simulink model "tensegrity_Val_like_sim"  (R2022b)
settings: Solver=VariableStepAuto  StartTime=0.0  StopTime=10.0  MaxStep=0.01  RelTol=1e-3
values from neighbouring files (symbols this model uses):
  a = 0.015    [parameters.m]
  bar_or_cable = 1    [parameters.m]
  bb = 1    [parameters.m]
  F1 = [pos1(1), pos1(2), pos1(3)]    [parameters.m]
  F2 = [pos1(1)+dist, pos1(2), pos1(3)]    [parameters.m]
  F3 = [pos1(1)+dist/2, pos1(2)+dist, pos1(3)]    [parameters.m]
  F4 = [pos2(1), pos2(2), pos2(3)]    [parameters.m]
  F5 = [pos2(1)+dist, pos2(2), pos2(3)]    [parameters.m]
  F6 = [pos2(1)+dist/2, pos2(2)+dist, pos2(3)]    [parameters.m]
  F7 = [pos3(1), pos3(2), pos3(3)]    [parameters.m]
  F8 = [pos3(1)+dist, pos3(2), pos3(3)]    [parameters.m]
  F9 = [pos3(1)+dist/2, pos3(2)+dist, pos3(3)]    [parameters.m]
  kk = 500    [parameters.m]
  l = [0.08 0.08 0.08 0.15]'    [parameters.m]
  lengths_0 = [lengths_0; l_i]    [tensegrity_Val_like.m]
  lf = 0.05*ones(9, 1)    [parameters.m]
undefined symbols (not defined in the file or in its folder): X, Y, Z
libraries: sm_lib x33, nesl_utility x31
settings Model: Creator=zavrel  LastModifiedBy=zavrel

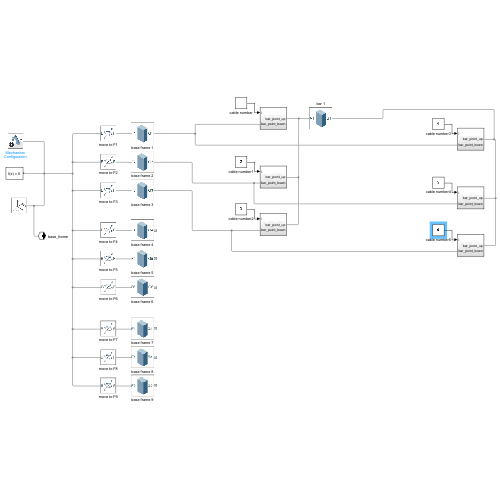
[thumbnail: Simulink's stored preview of the top-level diagram]
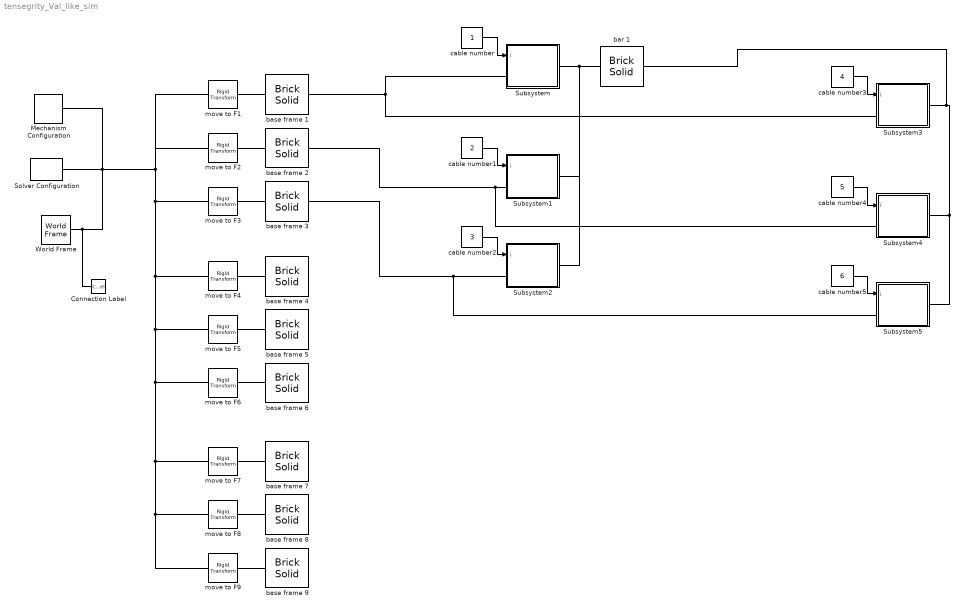
== system tensegrity_Val_like_sim ==
  Connection Label : ConnectionLabel  Label=base_frame
  Mechanism Configuration : sm_lib/Utilities/Mechanism Configuration  UniformGravity=Constant  GravityVector=[0 0 -9.80665]  GravityUnits=m/s^2  LinearizationDelta=0.001  JointModeTransitionNonlinearIterations=2
  Solver Configuration : nesl_utility/Solver Configuration  PhysicalDomain=network_engine_domain  SubClassName=solver  LeftPortType=input  RightPortType=generic  Tones=[]  Harmonics=[]  SimulateNoise=off  Profile=off  UseLocalSampling=off  EnableSwitchedLinearOptims=on  FrequencyDomain=off  UseCCode=off  RelTol=0.001  AbsTol=0.001  MinStep=1e-09  ToWorkspace=off  RevertToSquareIcSolve=off  NumHomotopyIterations=100  PhasorMode=off  PhasorModeNumHarmonics=1  ConsistencySolver=NEWTON_XTOL_AFTER_FTOL  IndexReductionMethod=DerivativeReplacement  DoDC=off  ResidualTolerance=1e-09  ConsistencyTolSource=GLOBAL  ConsistencyAbsTol=0.001  ConsistencyRelTol=0.001  ConsistencyTolFactor=0.001  UseLocalSolver=off  LocalSolverChoice=NE_BACKWARD_EULER_ADVANCER  ResolveIndetEquations=on  FunctionEvalNumThread=1  LocalSolverSampleTime=0.001  DoFixedCost=off  MaxNonlinIter=3  MaxModeIter=2  ComputeImpulses=off  ImpulseIterations=2  LinearAlgebra=auto  LinearAlgebraNumThread=0  EquationFormulation=NE_TIME_EF  DelaysMemoryBudget=1024  AutomaticFiltering=on  FilteringTimeConstant=0.001  PartitionStorageMethod=AS_NEEDED  PartitionMemoryBudget=1024  PartitionMethod=ROBUST
  Subsystem : Subsystem
  Subsystem1 : Subsystem
  Subsystem2 : Subsystem
  Subsystem3 : Subsystem
  Subsystem4 : Subsystem
  Subsystem5 : Subsystem
  World Frame : sm_lib/Frames and Transforms/World Frame
  bar 1 : sm_lib/Body Elements/Brick Solid  GraphicAmbientColor=[0.15 0.15 0.15 1.0]  BasedOnType=Density  BrickDimensions=[a a l(1)]  BrickDimensionUnits=m  CenterOfMass=[0 0 0]  CenterOfMassUnits=m  GraphicDiffuseColor=[0.5 0.5 0.5]  Density=rho  DensityUnits=kg/m^3  DoExposeReferenceFrame=off  GraphicEmissiveColor=[0.0 0.0 0.0 1.0]  ExportEntireGeometry=off  SerializedFrames=<Frames><Frame><Id>Frame1</Id><Value><Name>A1</Name><Origin><Source>GeometricFeature</Source><FeatureName>-z surface</FeatureName></Origin><PrimaryAxis><DefinedDirection>+Z</DefinedDirection><Source>ReferenceFrame</Source><SourceDirection>+Z</SourceDirection><FeatureName></FeatureName></PrimaryAxis><SecondaryAxis><DefinedDirection>+X</DefinedDirection><Source>ReferenceFrame</Source><SourceDirection>+X</SourceDirection><FeatureName></FeatureName></SecondaryAxis></Value></Frame><Frame><Id>Frame2</Id><Value><Name>B1</Name><Origin><Source>GeometricFeature</Source><FeatureName>+z surface</FeatureName></Origin><PrimaryAxis><DefinedDirection>+Z</DefinedDirection><Source>ReferenceFrame</Source><SourceDirection>+Z</SourceDirection><FeatureName></FeatureName></PrimaryAxis><SecondaryAxis><DefinedDirection>+X</DefinedDirection><Source>ReferenceFrame</Source><SourceDirection>+X</SourceDirection><FeatureName></FeatureName></SecondaryAxis></Value></Frame></Frames>  MarkerShape=Sphere  MarkerSize=10  GraphicType=FromGeometry  InertiaType=CalculateFromGeometry  Mass=1  MassUnits=kg  MomentsOfInertia=[1 1 1]  MomentsOfInertiaUnits=kg*m^2  GraphicOpacity=1.0  ProductsOfInertia=[0 0 0]  ProductsOfInertiaUnits=kg*m^2  GraphicShininess=75  GraphicSpecularColor=[0.5 0.5 0.5 1.0]  GraphicVisPropType=SimpleVisualProperties
  base frame 1 : sm_lib/Body Elements/Brick Solid  GraphicAmbientColor=[0.15 0.15 0.15 1.0]  BasedOnType=Density  BrickDimensions=[a a lf(1)]  BrickDimensionUnits=m  CenterOfMass=[0 0 0]  CenterOfMassUnits=m  GraphicDiffuseColor=[0.5 0.5 0.5]  Density=rho  DensityUnits=kg/m^3  DoExposeReferenceFrame=off  GraphicEmissiveColor=[0.0 0.0 0.0 1.0]  ExportEntireGeometry=off  SerializedFrames=<Frames><Frame><Id>Frame1</Id><Value><Name>F1</Name><Origin><Source>GeometricFeature</Source><FeatureName>-z surface</FeatureName></Origin><PrimaryAxis><DefinedDirection>+Z</DefinedDirection><Source>ReferenceFrame</Source><SourceDirection>+Z</SourceDirection><FeatureName></FeatureName></PrimaryAxis><SecondaryAxis><DefinedDirection>+X</DefinedDirection><Source>ReferenceFrame</Source><SourceDirection>+X</SourceDirection><FeatureName></FeatureName></SecondaryAxis></Value></Frame><Frame><Id>Frame2</Id><Value><Name>G1</Name><Origin><Source>GeometricFeature</Source><FeatureName>+z surface</FeatureName></Origin><PrimaryAxis><DefinedDirection>+Z</DefinedDirection><Source>ReferenceFrame</Source><SourceDirection>+Z</SourceDirection><FeatureName></FeatureName></PrimaryAxis><SecondaryAxis><DefinedDirection>+X</DefinedDirection><Source>ReferenceFrame</Source><SourceDirection>+X</SourceDirection><FeatureName></FeatureName></SecondaryAxis></Value></Frame></Frames>  MarkerShape=Sphere  MarkerSize=10  GraphicType=FromGeometry  InertiaType=CalculateFromGeometry  Mass=1  MassUnits=kg  MomentsOfInertia=[1 1 1]  MomentsOfInertiaUnits=kg*m^2  GraphicOpacity=1.0  ProductsOfInertia=[0 0 0]  ProductsOfInertiaUnits=kg*m^2  GraphicShininess=75  GraphicSpecularColor=[0.5 0.5 0.5 1.0]  GraphicVisPropType=SimpleVisualProperties
  base frame 2 : sm_lib/Body Elements/Brick Solid  GraphicAmbientColor=[0.15 0.15 0.15 1.0]  BasedOnType=Density  BrickDimensions=[a a lf(2)]  BrickDimensionUnits=m  CenterOfMass=[0 0 0]  CenterOfMassUnits=m  GraphicDiffuseColor=[0.5 0.5 0.5]  Density=rho  DensityUnits=kg/m^3  DoExposeReferenceFrame=off  GraphicEmissiveColor=[0.0 0.0 0.0 1.0]  ExportEntireGeometry=off  SerializedFrames=<Frames><Frame><Id>Frame1</Id><Value><Name>F2</Name><Origin><Source>GeometricFeature</Source><FeatureName>-z surface</FeatureName></Origin><PrimaryAxis><DefinedDirection>+Z</DefinedDirection><Source>ReferenceFrame</Source><SourceDirection>+Z</SourceDirection><FeatureName></FeatureName></PrimaryAxis><SecondaryAxis><DefinedDirection>+X</DefinedDirection><Source>ReferenceFrame</Source><SourceDirection>+X</SourceDirection><FeatureName></FeatureName></SecondaryAxis></Value></Frame><Frame><Id>Frame2</Id><Value><Name>G2</Name><Origin><Source>GeometricFeature</Source><FeatureName>+z surface</FeatureName></Origin><PrimaryAxis><DefinedDirection>+Z</DefinedDirection><Source>ReferenceFrame</Source><SourceDirection>+Z</SourceDirection><FeatureName></FeatureName></PrimaryAxis><SecondaryAxis><DefinedDirection>+X</DefinedDirection><Source>ReferenceFrame</Source><SourceDirection>+X</SourceDirection><FeatureName></FeatureName></SecondaryAxis></Value></Frame></Frames>  MarkerShape=Sphere  MarkerSize=10  GraphicType=FromGeometry  InertiaType=CalculateFromGeometry  Mass=1  MassUnits=kg  MomentsOfInertia=[1 1 1]  MomentsOfInertiaUnits=kg*m^2  GraphicOpacity=1.0  ProductsOfInertia=[0 0 0]  ProductsOfInertiaUnits=kg*m^2  GraphicShininess=75  GraphicSpecularColor=[0.5 0.5 0.5 1.0]  GraphicVisPropType=SimpleVisualProperties
  base frame 3 : sm_lib/Body Elements/Brick Solid  GraphicAmbientColor=[0.15 0.15 0.15 1.0]  BasedOnType=Density  BrickDimensions=[a a lf(3)]  BrickDimensionUnits=m  CenterOfMass=[0 0 0]  CenterOfMassUnits=m  GraphicDiffuseColor=[0.5 0.5 0.5]  Density=rho  DensityUnits=kg/m^3  DoExposeReferenceFrame=off  GraphicEmissiveColor=[0.0 0.0 0.0 1.0]  ExportEntireGeometry=off  SerializedFrames=<Frames><Frame><Id>Frame1</Id><Value><Name>F3</Name><Origin><Source>GeometricFeature</Source><FeatureName>-z surface</FeatureName></Origin><PrimaryAxis><DefinedDirection>+Z</DefinedDirection><Source>ReferenceFrame</Source><SourceDirection>+Z</SourceDirection><FeatureName></FeatureName></PrimaryAxis><SecondaryAxis><DefinedDirection>+X</DefinedDirection><Source>ReferenceFrame</Source><SourceDirection>+X</SourceDirection><FeatureName></FeatureName></SecondaryAxis></Value></Frame><Frame><Id>Frame2</Id><Value><Name>G3</Name><Origin><Source>GeometricFeature</Source><FeatureName>+z surface</FeatureName></Origin><PrimaryAxis><DefinedDirection>+Z</DefinedDirection><Source>ReferenceFrame</Source><SourceDirection>+Z</SourceDirection><FeatureName></FeatureName></PrimaryAxis><SecondaryAxis><DefinedDirection>+X</DefinedDirection><Source>ReferenceFrame</Source><SourceDirection>+X</SourceDirection><FeatureName></FeatureName></SecondaryAxis></Value></Frame></Frames>  MarkerShape=Sphere  MarkerSize=10  GraphicType=FromGeometry  InertiaType=CalculateFromGeometry  Mass=1  MassUnits=kg  MomentsOfInertia=[1 1 1]  MomentsOfInertiaUnits=kg*m^2  GraphicOpacity=1.0  ProductsOfInertia=[0 0 0]  ProductsOfInertiaUnits=kg*m^2  GraphicShininess=75  GraphicSpecularColor=[0.5 0.5 0.5 1.0]  GraphicVisPropType=SimpleVisualProperties
  base frame 4 : sm_lib/Body Elements/Brick Solid  GraphicAmbientColor=[0.15 0.15 0.15 1.0]  BasedOnType=Density  BrickDimensions=[a a lf(4)]  BrickDimensionUnits=m  CenterOfMass=[0 0 0]  CenterOfMassUnits=m  GraphicDiffuseColor=[0.5 0.5 0.5]  Density=rho  DensityUnits=kg/m^3  DoExposeReferenceFrame=off  GraphicEmissiveColor=[0.0 0.0 0.0 1.0]  ExportEntireGeometry=off  SerializedFrames=<Frames><Frame><Id>Frame1</Id><Value><Name>F4</Name><Origin><Source>GeometricFeature</Source><FeatureName>-z surface</FeatureName></Origin><PrimaryAxis><DefinedDirection>+Z</DefinedDirection><Source>ReferenceFrame</Source><SourceDirection>+Z</SourceDirection><FeatureName></FeatureName></PrimaryAxis><SecondaryAxis><DefinedDirection>+X</DefinedDirection><Source>ReferenceFrame</Source><SourceDirection>+X</SourceDirection><FeatureName></FeatureName></SecondaryAxis></Value></Frame><Frame><Id>Frame2</Id><Value><Name>G4</Name><Origin><Source>GeometricFeature</Source><FeatureName>+z surface</FeatureName></Origin><PrimaryAxis><DefinedDirection>+Z</DefinedDirection><Source>ReferenceFrame</Source><SourceDirection>+Z</SourceDirection><FeatureName></FeatureName></PrimaryAxis><SecondaryAxis><DefinedDirection>+X</DefinedDirection><Source>ReferenceFrame</Source><SourceDirection>+X</SourceDirection><FeatureName></FeatureName></SecondaryAxis></Value></Frame></Frames>  MarkerShape=Sphere  MarkerSize=10  GraphicType=FromGeometry  InertiaType=CalculateFromGeometry  Mass=1  MassUnits=kg  MomentsOfInertia=[1 1 1]  MomentsOfInertiaUnits=kg*m^2  GraphicOpacity=1.0  ProductsOfInertia=[0 0 0]  ProductsOfInertiaUnits=kg*m^2  GraphicShininess=75  GraphicSpecularColor=[0.5 0.5 0.5 1.0]  GraphicVisPropType=SimpleVisualProperties
  base frame 5 : sm_lib/Body Elements/Brick Solid  GraphicAmbientColor=[0.15 0.15 0.15 1.0]  BasedOnType=Density  BrickDimensions=[a a lf(5)]  BrickDimensionUnits=m  CenterOfMass=[0 0 0]  CenterOfMassUnits=m  GraphicDiffuseColor=[0.5 0.5 0.5]  Density=rho  DensityUnits=kg/m^3  DoExposeReferenceFrame=off  GraphicEmissiveColor=[0.0 0.0 0.0 1.0]  ExportEntireGeometry=off  SerializedFrames=<Frames><Frame><Id>Frame1</Id><Value><Name>F5</Name><Origin><Source>GeometricFeature</Source><FeatureName>-z surface</FeatureName></Origin><PrimaryAxis><DefinedDirection>+Z</DefinedDirection><Source>ReferenceFrame</Source><SourceDirection>+Z</SourceDirection><FeatureName></FeatureName></PrimaryAxis><SecondaryAxis><DefinedDirection>+X</DefinedDirection><Source>ReferenceFrame</Source><SourceDirection>+X</SourceDirection><FeatureName></FeatureName></SecondaryAxis></Value></Frame><Frame><Id>Frame2</Id><Value><Name>G5</Name><Origin><Source>GeometricFeature</Source><FeatureName>+z surface</FeatureName></Origin><PrimaryAxis><DefinedDirection>+Z</DefinedDirection><Source>ReferenceFrame</Source><SourceDirection>+Z</SourceDirection><FeatureName></FeatureName></PrimaryAxis><SecondaryAxis><DefinedDirection>+X</DefinedDirection><Source>ReferenceFrame</Source><SourceDirection>+X</SourceDirection><FeatureName></FeatureName></SecondaryAxis></Value></Frame></Frames>  MarkerShape=Sphere  MarkerSize=10  GraphicType=FromGeometry  InertiaType=CalculateFromGeometry  Mass=1  MassUnits=kg  MomentsOfInertia=[1 1 1]  MomentsOfInertiaUnits=kg*m^2  GraphicOpacity=1.0  ProductsOfInertia=[0 0 0]  ProductsOfInertiaUnits=kg*m^2  GraphicShininess=75  GraphicSpecularColor=[0.5 0.5 0.5 1.0]  GraphicVisPropType=SimpleVisualProperties
  base frame 6 : sm_lib/Body Elements/Brick Solid  GraphicAmbientColor=[0.15 0.15 0.15 1.0]  BasedOnType=Density  BrickDimensions=[a a lf(6)]  BrickDimensionUnits=m  CenterOfMass=[0 0 0]  CenterOfMassUnits=m  GraphicDiffuseColor=[0.5 0.5 0.5]  Density=rho  DensityUnits=kg/m^3  DoExposeReferenceFrame=off  GraphicEmissiveColor=[0.0 0.0 0.0 1.0]  ExportEntireGeometry=off  SerializedFrames=<Frames><Frame><Id>Frame1</Id><Value><Name>F6</Name><Origin><Source>GeometricFeature</Source><FeatureName>-z surface</FeatureName></Origin><PrimaryAxis><DefinedDirection>+Z</DefinedDirection><Source>ReferenceFrame</Source><SourceDirection>+Z</SourceDirection><FeatureName></FeatureName></PrimaryAxis><SecondaryAxis><DefinedDirection>+X</DefinedDirection><Source>ReferenceFrame</Source><SourceDirection>+X</SourceDirection><FeatureName></FeatureName></SecondaryAxis></Value></Frame><Frame><Id>Frame2</Id><Value><Name>G6</Name><Origin><Source>GeometricFeature</Source><FeatureName>+z surface</FeatureName></Origin><PrimaryAxis><DefinedDirection>+Z</DefinedDirection><Source>ReferenceFrame</Source><SourceDirection>+Z</SourceDirection><FeatureName></FeatureName></PrimaryAxis><SecondaryAxis><DefinedDirection>+X</DefinedDirection><Source>ReferenceFrame</Source><SourceDirection>+X</SourceDirection><FeatureName></FeatureName></SecondaryAxis></Value></Frame></Frames>  MarkerShape=Sphere  MarkerSize=10  GraphicType=FromGeometry  InertiaType=CalculateFromGeometry  Mass=1  MassUnits=kg  MomentsOfInertia=[1 1 1]  MomentsOfInertiaUnits=kg*m^2  GraphicOpacity=1.0  ProductsOfInertia=[0 0 0]  ProductsOfInertiaUnits=kg*m^2  GraphicShininess=75  GraphicSpecularColor=[0.5 0.5 0.5 1.0]  GraphicVisPropType=SimpleVisualProperties
  base frame 7 : sm_lib/Body Elements/Brick Solid  GraphicAmbientColor=[0.15 0.15 0.15 1.0]  BasedOnType=Density  BrickDimensions=[a a lf(1)]  BrickDimensionUnits=m  CenterOfMass=[0 0 0]  CenterOfMassUnits=m  GraphicDiffuseColor=[0.5 0.5 0.5]  Density=rho  DensityUnits=kg/m^3  DoExposeReferenceFrame=off  GraphicEmissiveColor=[0.0 0.0 0.0 1.0]  ExportEntireGeometry=off  SerializedFrames=<Frames><Frame><Id>Frame1</Id><Value><Name>F1</Name><Origin><Source>GeometricFeature</Source><FeatureName>-z surface</FeatureName></Origin><PrimaryAxis><DefinedDirection>+Z</DefinedDirection><Source>ReferenceFrame</Source><SourceDirection>+Z</SourceDirection><FeatureName></FeatureName></PrimaryAxis><SecondaryAxis><DefinedDirection>+X</DefinedDirection><Source>ReferenceFrame</Source><SourceDirection>+X</SourceDirection><FeatureName></FeatureName></SecondaryAxis></Value></Frame><Frame><Id>Frame2</Id><Value><Name>G1</Name><Origin><Source>GeometricFeature</Source><FeatureName>+z surface</FeatureName></Origin><PrimaryAxis><DefinedDirection>+Z</DefinedDirection><Source>ReferenceFrame</Source><SourceDirection>+Z</SourceDirection><FeatureName></FeatureName></PrimaryAxis><SecondaryAxis><DefinedDirection>+X</DefinedDirection><Source>ReferenceFrame</Source><SourceDirection>+X</SourceDirection><FeatureName></FeatureName></SecondaryAxis></Value></Frame></Frames>  MarkerShape=Sphere  MarkerSize=10  GraphicType=FromGeometry  InertiaType=CalculateFromGeometry  Mass=1  MassUnits=kg  MomentsOfInertia=[1 1 1]  MomentsOfInertiaUnits=kg*m^2  GraphicOpacity=1.0  ProductsOfInertia=[0 0 0]  ProductsOfInertiaUnits=kg*m^2  GraphicShininess=75  GraphicSpecularColor=[0.5 0.5 0.5 1.0]  GraphicVisPropType=SimpleVisualProperties
  base frame 8 : sm_lib/Body Elements/Brick Solid  GraphicAmbientColor=[0.15 0.15 0.15 1.0]  BasedOnType=Density  BrickDimensions=[a a lf(1)]  BrickDimensionUnits=m  CenterOfMass=[0 0 0]  CenterOfMassUnits=m  GraphicDiffuseColor=[0.5 0.5 0.5]  Density=rho  DensityUnits=kg/m^3  DoExposeReferenceFrame=off  GraphicEmissiveColor=[0.0 0.0 0.0 1.0]  ExportEntireGeometry=off  SerializedFrames=<Frames><Frame><Id>Frame1</Id><Value><Name>F1</Name><Origin><Source>GeometricFeature</Source><FeatureName>-z surface</FeatureName></Origin><PrimaryAxis><DefinedDirection>+Z</DefinedDirection><Source>ReferenceFrame</Source><SourceDirection>+Z</SourceDirection><FeatureName></FeatureName></PrimaryAxis><SecondaryAxis><DefinedDirection>+X</DefinedDirection><Source>ReferenceFrame</Source><SourceDirection>+X</SourceDirection><FeatureName></FeatureName></SecondaryAxis></Value></Frame><Frame><Id>Frame2</Id><Value><Name>G1</Name><Origin><Source>GeometricFeature</Source><FeatureName>+z surface</FeatureName></Origin><PrimaryAxis><DefinedDirection>+Z</DefinedDirection><Source>ReferenceFrame</Source><SourceDirection>+Z</SourceDirection><FeatureName></FeatureName></PrimaryAxis><SecondaryAxis><DefinedDirection>+X</DefinedDirection><Source>ReferenceFrame</Source><SourceDirection>+X</SourceDirection><FeatureName></FeatureName></SecondaryAxis></Value></Frame></Frames>  MarkerShape=Sphere  MarkerSize=10  GraphicType=FromGeometry  InertiaType=CalculateFromGeometry  Mass=1  MassUnits=kg  MomentsOfInertia=[1 1 1]  MomentsOfInertiaUnits=kg*m^2  GraphicOpacity=1.0  ProductsOfInertia=[0 0 0]  ProductsOfInertiaUnits=kg*m^2  GraphicShininess=75  GraphicSpecularColor=[0.5 0.5 0.5 1.0]  GraphicVisPropType=SimpleVisualProperties
  base frame 9 : sm_lib/Body Elements/Brick Solid  GraphicAmbientColor=[0.15 0.15 0.15 1.0]  BasedOnType=Density  BrickDimensions=[a a lf(9)]  BrickDimensionUnits=m  CenterOfMass=[0 0 0]  CenterOfMassUnits=m  GraphicDiffuseColor=[0.5 0.5 0.5]  Density=rho  DensityUnits=kg/m^3  DoExposeReferenceFrame=off  GraphicEmissiveColor=[0.0 0.0 0.0 1.0]  ExportEntireGeometry=off  SerializedFrames=<Frames><Frame><Id>Frame1</Id><Value><Name>F9</Name><Origin><Source>GeometricFeature</Source><FeatureName>-z surface</FeatureName></Origin><PrimaryAxis><DefinedDirection>+Z</DefinedDirection><Source>ReferenceFrame</Source><SourceDirection>+Z</SourceDirection><FeatureName></FeatureName></PrimaryAxis><SecondaryAxis><DefinedDirection>+X</DefinedDirection><Source>ReferenceFrame</Source><SourceDirection>+X</SourceDirection><FeatureName></FeatureName></SecondaryAxis></Value></Frame><Frame><Id>Frame2</Id><Value><Name>G9</Name><Origin><Source>GeometricFeature</Source><FeatureName>+z surface</FeatureName></Origin><PrimaryAxis><DefinedDirection>+Z</DefinedDirection><Source>ReferenceFrame</Source><SourceDirection>+Z</SourceDirection><FeatureName></FeatureName></PrimaryAxis><SecondaryAxis><DefinedDirection>+X</DefinedDirection><Source>ReferenceFrame</Source><SourceDirection>+X</SourceDirection><FeatureName></FeatureName></SecondaryAxis></Value></Frame></Frames>  MarkerShape=Sphere  MarkerSize=10  GraphicType=FromGeometry  InertiaType=CalculateFromGeometry  Mass=1  MassUnits=kg  MomentsOfInertia=[1 1 1]  MomentsOfInertiaUnits=kg*m^2  GraphicOpacity=1.0  ProductsOfInertia=[0 0 0]  ProductsOfInertiaUnits=kg*m^2  GraphicShininess=75  GraphicSpecularColor=[0.5 0.5 0.5 1.0]  GraphicVisPropType=SimpleVisualProperties
  cable number : Constant
  cable number1 : Constant  Value=2
  cable number2 : Constant  Value=3
  cable number3 : Constant  Value=4
  cable number4 : Constant  Value=5
  cable number5 : Constant  Value=6
  move to F1 : sm_lib/Frames and Transforms/Rigid Transform  TranslationMethod=Cartesian  TranslationStandardOffset=0  TranslationLengthUnit=m  TranslationStandardAxis=+Z  TranslationCartesianOffset=[F1(1) F1(2) F1(3)]  TranslationROffset=0  TranslationROffsetUnits=m  TranslationZOffset=0  TranslationZOffsetUnits=m  TranslationThetaOffset=0  TranslationThetaOffsetUnits=deg  RotationMethod=None  RotationAngleUnits=deg  RotationStandardAxis=+Z  RotationAngle=0.0  RotationArbitraryAxis=[0 0 1]  FollAlignAxisA=+X  BaseAlignAxisA=+Y  FollAlignAxisB=+Y  BaseAlignAxisB=+Z  RotationSequenceAxes=FollowerAxes  RotationSequence=XYX  RotationSequenceAngles=[0 0 0]  RotationSequenceAnglesUnits=deg  RotationMatrix=[1 0 0; 0 1 0; 0 0 1]  Quaternion=[1 0 0 0]
  move to F2 : sm_lib/Frames and Transforms/Rigid Transform  TranslationMethod=Cartesian  TranslationStandardOffset=0  TranslationLengthUnit=m  TranslationStandardAxis=+Z  TranslationCartesianOffset=[F2(1) F2(2) F2(3)]  TranslationROffset=0  TranslationROffsetUnits=m  TranslationZOffset=0  TranslationZOffsetUnits=m  TranslationThetaOffset=0  TranslationThetaOffsetUnits=deg  RotationMethod=None  RotationAngleUnits=deg  RotationStandardAxis=+Z  RotationAngle=0.0  RotationArbitraryAxis=[0 0 1]  FollAlignAxisA=+X  BaseAlignAxisA=+Y  FollAlignAxisB=+Y  BaseAlignAxisB=+Z  RotationSequenceAxes=FollowerAxes  RotationSequence=XYX  RotationSequenceAngles=[0 0 0]  RotationSequenceAnglesUnits=deg  RotationMatrix=[1 0 0; 0 1 0; 0 0 1]  Quaternion=[1 0 0 0]
  move to F3 : sm_lib/Frames and Transforms/Rigid Transform  TranslationMethod=Cartesian  TranslationStandardOffset=0  TranslationLengthUnit=m  TranslationStandardAxis=+Z  TranslationCartesianOffset=[F3(1) F3(2) F3(3)]  TranslationROffset=0  TranslationROffsetUnits=m  TranslationZOffset=0  TranslationZOffsetUnits=m  TranslationThetaOffset=0  TranslationThetaOffsetUnits=deg  RotationMethod=None  RotationAngleUnits=deg  RotationStandardAxis=+Z  RotationAngle=0.0  RotationArbitraryAxis=[0 0 1]  FollAlignAxisA=+X  BaseAlignAxisA=+Y  FollAlignAxisB=+Y  BaseAlignAxisB=+Z  RotationSequenceAxes=FollowerAxes  RotationSequence=XYX  RotationSequenceAngles=[0 0 0]  RotationSequenceAnglesUnits=deg  RotationMatrix=[1 0 0; 0 1 0; 0 0 1]  Quaternion=[1 0 0 0]
  move to F4 : sm_lib/Frames and Transforms/Rigid Transform  TranslationMethod=Cartesian  TranslationStandardOffset=0  TranslationLengthUnit=m  TranslationStandardAxis=+Z  TranslationCartesianOffset=[F4(1) F4(2) F4(3)]  TranslationROffset=0  TranslationROffsetUnits=m  TranslationZOffset=0  TranslationZOffsetUnits=m  TranslationThetaOffset=0  TranslationThetaOffsetUnits=deg  RotationMethod=None  RotationAngleUnits=deg  RotationStandardAxis=+Z  RotationAngle=0.0  RotationArbitraryAxis=[0 0 1]  FollAlignAxisA=+X  BaseAlignAxisA=+Y  FollAlignAxisB=+Y  BaseAlignAxisB=+Z  RotationSequenceAxes=FollowerAxes  RotationSequence=XYX  RotationSequenceAngles=[0 0 0]  RotationSequenceAnglesUnits=deg  RotationMatrix=[1 0 0; 0 1 0; 0 0 1]  Quaternion=[1 0 0 0]
  move to F5 : sm_lib/Frames and Transforms/Rigid Transform  TranslationMethod=Cartesian  TranslationStandardOffset=0  TranslationLengthUnit=m  TranslationStandardAxis=+Z  TranslationCartesianOffset=[F5(1) F5(2) F5(3)]  TranslationROffset=0  TranslationROffsetUnits=m  TranslationZOffset=0  TranslationZOffsetUnits=m  TranslationThetaOffset=0  TranslationThetaOffsetUnits=deg  RotationMethod=None  RotationAngleUnits=deg  RotationStandardAxis=+Z  RotationAngle=0.0  RotationArbitraryAxis=[0 0 1]  FollAlignAxisA=+X  BaseAlignAxisA=+Y  FollAlignAxisB=+Y  BaseAlignAxisB=+Z  RotationSequenceAxes=FollowerAxes  RotationSequence=XYX  RotationSequenceAngles=[0 0 0]  RotationSequenceAnglesUnits=deg  RotationMatrix=[1 0 0; 0 1 0; 0 0 1]  Quaternion=[1 0 0 0]
  move to F6 : sm_lib/Frames and Transforms/Rigid Transform  TranslationMethod=Cartesian  TranslationStandardOffset=0  TranslationLengthUnit=m  TranslationStandardAxis=+Z  TranslationCartesianOffset=[F6(1) F6(2) F6(3)]  TranslationROffset=0  TranslationROffsetUnits=m  TranslationZOffset=0  TranslationZOffsetUnits=m  TranslationThetaOffset=0  TranslationThetaOffsetUnits=deg  RotationMethod=None  RotationAngleUnits=deg  RotationStandardAxis=+Z  RotationAngle=0.0  RotationArbitraryAxis=[0 0 1]  FollAlignAxisA=+X  BaseAlignAxisA=+Y  FollAlignAxisB=+Y  BaseAlignAxisB=+Z  RotationSequenceAxes=FollowerAxes  RotationSequence=XYX  RotationSequenceAngles=[0 0 0]  RotationSequenceAnglesUnits=deg  RotationMatrix=[1 0 0; 0 1 0; 0 0 1]  Quaternion=[1 0 0 0]
  move to F7 : sm_lib/Frames and Transforms/Rigid Transform  TranslationMethod=Cartesian  TranslationStandardOffset=0  TranslationLengthUnit=m  TranslationStandardAxis=+Z  TranslationCartesianOffset=[F7(1) F7(2) F7(3)]  TranslationROffset=0  TranslationROffsetUnits=m  TranslationZOffset=0  TranslationZOffsetUnits=m  TranslationThetaOffset=0  TranslationThetaOffsetUnits=deg  RotationMethod=None  RotationAngleUnits=deg  RotationStandardAxis=+Z  RotationAngle=0.0  RotationArbitraryAxis=[0 0 1]  FollAlignAxisA=+X  BaseAlignAxisA=+Y  FollAlignAxisB=+Y  BaseAlignAxisB=+Z  RotationSequenceAxes=FollowerAxes  RotationSequence=XYX  RotationSequenceAngles=[0 0 0]  RotationSequenceAnglesUnits=deg  RotationMatrix=[1 0 0; 0 1 0; 0 0 1]  Quaternion=[1 0 0 0]
  move to F8 : sm_lib/Frames and Transforms/Rigid Transform  TranslationMethod=Cartesian  TranslationStandardOffset=0  TranslationLengthUnit=m  TranslationStandardAxis=+Z  TranslationCartesianOffset=[F8(1) F8(2) F8(3)]  TranslationROffset=0  TranslationROffsetUnits=m  TranslationZOffset=0  TranslationZOffsetUnits=m  TranslationThetaOffset=0  TranslationThetaOffsetUnits=deg  RotationMethod=None  RotationAngleUnits=deg  RotationStandardAxis=+Z  RotationAngle=0.0  RotationArbitraryAxis=[0 0 1]  FollAlignAxisA=+X  BaseAlignAxisA=+Y  FollAlignAxisB=+Y  BaseAlignAxisB=+Z  RotationSequenceAxes=FollowerAxes  RotationSequence=XYX  RotationSequenceAngles=[0 0 0]  RotationSequenceAnglesUnits=deg  RotationMatrix=[1 0 0; 0 1 0; 0 0 1]  Quaternion=[1 0 0 0]
  move to F9 : sm_lib/Frames and Transforms/Rigid Transform  TranslationMethod=Cartesian  TranslationStandardOffset=0  TranslationLengthUnit=m  TranslationStandardAxis=+Z  TranslationCartesianOffset=[F9(1) F9(2) F9(3)]  TranslationROffset=0  TranslationROffsetUnits=m  TranslationZOffset=0  TranslationZOffsetUnits=m  TranslationThetaOffset=0  TranslationThetaOffsetUnits=deg  RotationMethod=None  RotationAngleUnits=deg  RotationStandardAxis=+Z  RotationAngle=0.0  RotationArbitraryAxis=[0 0 1]  FollAlignAxisA=+X  BaseAlignAxisA=+Y  FollAlignAxisB=+Y  BaseAlignAxisB=+Z  RotationSequenceAxes=FollowerAxes  RotationSequence=XYX  RotationSequenceAngles=[0 0 0]  RotationSequenceAnglesUnits=deg  RotationMatrix=[1 0 0; 0 1 0; 0 0 1]  Quaternion=[1 0 0 0]
  wires:
  cable number/1 -> Subsystem/1(i)
  cable number1/1 -> Subsystem1/1(i)
  cable number2/1 -> Subsystem2/1(i)
  cable number4/1 -> Subsystem4/1(i)
  cable number3/1 -> Subsystem3/1(i)
  cable number5/1 -> Subsystem5/1(i)
  connections:
  base frame 1/LConn1 -- move to F1/RConn1
  base frame 2/LConn1 -- move to F2/RConn1
  base frame 3/LConn1 -- move to F3/RConn1
  base frame 6/LConn1 -- move to F6/RConn1
  base frame 5/LConn1 -- move to F5/RConn1
  base frame 4/LConn1 -- move to F4/RConn1
  base frame 7/LConn1 -- move to F7/RConn1
  base frame 8/LConn1 -- move to F8/RConn1
  base frame 9/LConn1 -- move to F9/RConn1
  Mechanism Configuration/RConn1 -- move to F2/LConn1 -- move to F1/LConn1 -- move to F3/LConn1 -- move to F4/LConn1 -- move to F5/LConn1 -- move to F6/LConn1 -- move to F7/LConn1 -- move to F8/LConn1 -- move to F9/LConn1 -- Connection Label/LConn1 -- World Frame/RConn1 -- Solver Configuration/RConn1
  Subsystem/RConn1 -- Subsystem2/RConn1 -- Subsystem1/RConn1 -- bar 1/LConn1
  base frame 1/RConn1 -- Subsystem/LConn1 -- Subsystem3/LConn1
  Subsystem1/LConn1 -- base frame 2/RConn1 -- Subsystem4/LConn1
  Subsystem2/LConn1 -- Subsystem5/LConn1 -- base frame 3/RConn1
  Subsystem4/RConn1 -- bar 1/RConn1 -- Subsystem3/RConn1 -- Subsystem5/RConn1

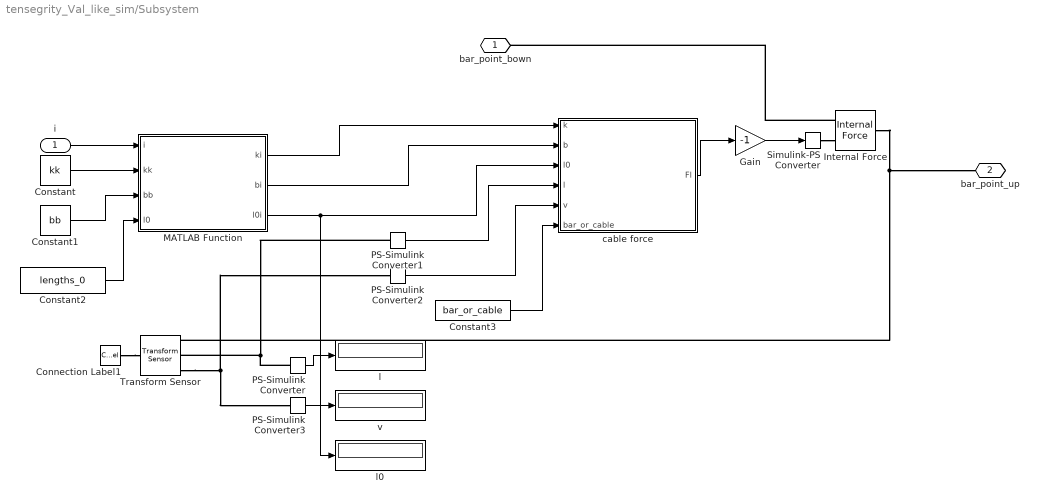
== system tensegrity_Val_like_sim/Subsystem ==
  i : Inport
  Connection Label1 : ConnectionLabel  Label=base_frame
  Constant : Constant  Value=kk
  Constant1 : Constant  Value=bb
  Constant2 : Constant  Value=lengths_0
  Constant3 : Constant  Value=bar_or_cable
  Gain : Gain  Gain=-1
  Internal Force : sm_lib/Forces and Torques/Internal Force
  MATLAB Function : MATLAB Function  TreatAsAtomicUnit=on
  PS-Simulink Converter{,1..3} (4 alike) : nesl_utility/PS-Simulink Converter  PhysicalDomain=network_engine_domain  SubClassName=ps_output  LeftPortType=input  RightPortType=output  PseudoPeriodic=off  Frequencies=[]  VectorFormat=inherit  Unit=inherit  AffineConversion=off
  Simulink-PS Converter : nesl_utility/Simulink-PS Converter  PhysicalDomain=network_engine_domain  SubClassName=ps_input  LeftPortType=input  RightPortType=output  PseudoPeriodic=off  Frequencies=[]  NoiseDistribution=none  NoiseParameters=[]  Unit=1  AffineConversion=off  FilteringAndDerivatives=provide  SimscapeFilterOrder=1  InputFilterTimeConstant=0.001  UdotUserProvided=0
  Transform Sensor : sm_lib/Frames and Transforms/Transform Sensor  MeasurementFrame=World  SenseAngle=off  SenseAxis=off  SenseQ=off  SenseR=off  SenseRotationSequence=off  RotationSequence=XYX  SenseOmegaX=off  SenseOmegaY=off  SenseOmegaZ=off  SenseQDot=off  SenseRDot=off  SenseAlphaX=off  SenseAlphaY=off  SenseAlphaZ=off  SenseQDDot=off  SenseRDDot=off  SenseX=off  SenseY=off  SenseZ=off  SenseRad=off  SenseAzim=off  SenseDist=on  SenseInc=off  SenseXDot=off  SenseYDot=off  SenseZDot=off  SenseRadDot=off  SenseAzimDot=off  SenseDistDot=on  SenseIncDot=off  SenseXDDot=off  SenseYDDot=off  SenseZDDot=off  SenseRadDDot=off  SenseAzimDDot=off  SenseDistDDot=off  SenseIncDDot=off
  cable force : MATLAB Function  TreatAsAtomicUnit=on
  l : Display
  l0 : Display
  v : Display
  bar_point_bown : PMIOPort  Side=Left
  bar_point_up : PMIOPort  Port=2  Side=Right
  wires:
  cable force/1(Fl) -> Gain/1
  PS-Simulink Converter/1 -> l/1
  Constant2/1 -> MATLAB Function/4(l0)
  MATLAB Function/2(bi) -> cable force/2(b)
  Constant1/1 -> MATLAB Function/3(bb)
  Constant/1 -> MATLAB Function/2(kk)
  MATLAB Function/1(ki) -> cable force/1(k)
  PS-Simulink Converter1/1 -> cable force/4(l)
  MATLAB Function/3(l0i) -> l0/1, cable force/3(l0)
  i/1 -> MATLAB Function/1(i)
  Constant3/1 -> cable force/6(bar_or_cable)
  Gain/1 -> Simulink-PS Converter/1
  PS-Simulink Converter2/1 -> cable force/5(v)
  PS-Simulink Converter3/1 -> v/1
  connections:
  Internal Force/LConn1 -- bar_point_bown/RConn1
  PS-Simulink Converter/LConn1 -- PS-Simulink Converter1/LConn1 -- Transform Sensor/RConn2
  Simulink-PS Converter/RConn1 -- Internal Force/LConn2
  Internal Force/RConn1 -- bar_point_up/RConn1 -- Transform Sensor/RConn1
  Connection Label1/LConn1 -- Transform Sensor/LConn1
  Transform Sensor/RConn3 -- PS-Simulink Converter3/LConn1 -- PS-Simulink Converter2/LConn1

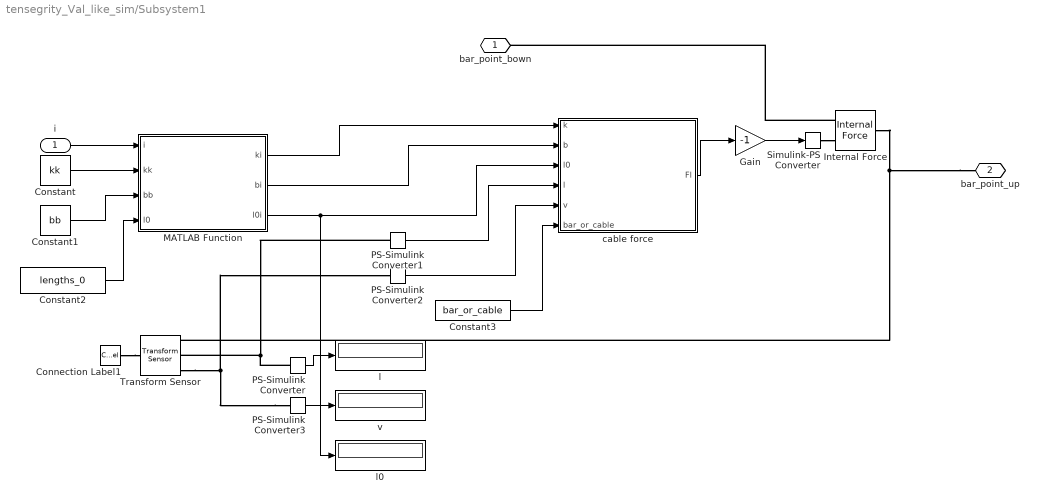
== system tensegrity_Val_like_sim/Subsystem1 ==
  i : Inport
  Connection Label1 : ConnectionLabel  Label=base_frame
  Constant : Constant  Value=kk
  Constant1 : Constant  Value=bb
  Constant2 : Constant  Value=lengths_0
  Constant3 : Constant  Value=bar_or_cable
  Gain : Gain  Gain=-1
  Internal Force : sm_lib/Forces and Torques/Internal Force
  MATLAB Function : MATLAB Function  TreatAsAtomicUnit=on
  PS-Simulink Converter{,1..3} (4 alike) : nesl_utility/PS-Simulink Converter  PhysicalDomain=network_engine_domain  SubClassName=ps_output  LeftPortType=input  RightPortType=output  PseudoPeriodic=off  Frequencies=[]  VectorFormat=inherit  Unit=inherit  AffineConversion=off
  Simulink-PS Converter : nesl_utility/Simulink-PS Converter  PhysicalDomain=network_engine_domain  SubClassName=ps_input  LeftPortType=input  RightPortType=output  PseudoPeriodic=off  Frequencies=[]  NoiseDistribution=none  NoiseParameters=[]  Unit=1  AffineConversion=off  FilteringAndDerivatives=provide  SimscapeFilterOrder=1  InputFilterTimeConstant=0.001  UdotUserProvided=0
  Transform Sensor : sm_lib/Frames and Transforms/Transform Sensor  MeasurementFrame=World  SenseAngle=off  SenseAxis=off  SenseQ=off  SenseR=off  SenseRotationSequence=off  RotationSequence=XYX  SenseOmegaX=off  SenseOmegaY=off  SenseOmegaZ=off  SenseQDot=off  SenseRDot=off  SenseAlphaX=off  SenseAlphaY=off  SenseAlphaZ=off  SenseQDDot=off  SenseRDDot=off  SenseX=off  SenseY=off  SenseZ=off  SenseRad=off  SenseAzim=off  SenseDist=on  SenseInc=off  SenseXDot=off  SenseYDot=off  SenseZDot=off  SenseRadDot=off  SenseAzimDot=off  SenseDistDot=on  SenseIncDot=off  SenseXDDot=off  SenseYDDot=off  SenseZDDot=off  SenseRadDDot=off  SenseAzimDDot=off  SenseDistDDot=off  SenseIncDDot=off
  cable force : MATLAB Function  TreatAsAtomicUnit=on
  l : Display
  l0 : Display
  v : Display
  bar_point_bown : PMIOPort  Side=Left
  bar_point_up : PMIOPort  Port=2  Side=Right
  wires:
  PS-Simulink Converter3/1 -> v/1
  PS-Simulink Converter2/1 -> cable force/5(v)
  Gain/1 -> Simulink-PS Converter/1
  Constant3/1 -> cable force/6(bar_or_cable)
  i/1 -> MATLAB Function/1(i)
  MATLAB Function/3(l0i) -> cable force/3(l0), l0/1
  PS-Simulink Converter1/1 -> cable force/4(l)
  MATLAB Function/1(ki) -> cable force/1(k)
  Constant/1 -> MATLAB Function/2(kk)
  Constant1/1 -> MATLAB Function/3(bb)
  MATLAB Function/2(bi) -> cable force/2(b)
  Constant2/1 -> MATLAB Function/4(l0)
  PS-Simulink Converter/1 -> l/1
  cable force/1(Fl) -> Gain/1
  connections:
  PS-Simulink Converter3/LConn1 -- Transform Sensor/RConn3 -- PS-Simulink Converter2/LConn1
  Connection Label1/LConn1 -- Transform Sensor/LConn1
  bar_point_up/RConn1 -- Transform Sensor/RConn1 -- Internal Force/RConn1
  Simulink-PS Converter/RConn1 -- Internal Force/LConn2
  PS-Simulink Converter1/LConn1 -- Transform Sensor/RConn2 -- PS-Simulink Converter/LConn1
  Internal Force/LConn1 -- bar_point_bown/RConn1

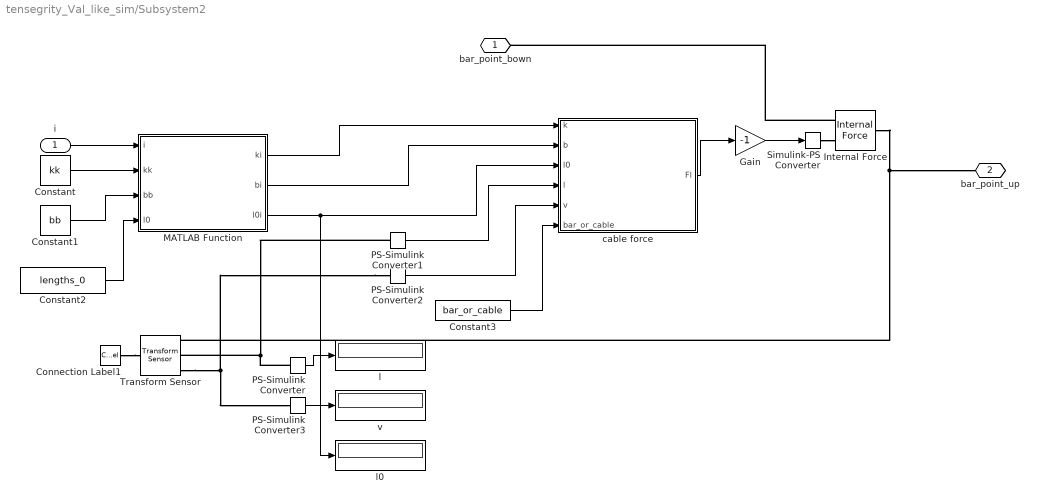
== system tensegrity_Val_like_sim/Subsystem2 ==
  i : Inport
  Connection Label1 : ConnectionLabel  Label=base_frame
  Constant : Constant  Value=kk
  Constant1 : Constant  Value=bb
  Constant2 : Constant  Value=lengths_0
  Constant3 : Constant  Value=bar_or_cable
  Gain : Gain  Gain=-1
  Internal Force : sm_lib/Forces and Torques/Internal Force
  MATLAB Function : MATLAB Function  TreatAsAtomicUnit=on
  PS-Simulink Converter{,1..3} (4 alike) : nesl_utility/PS-Simulink Converter  PhysicalDomain=network_engine_domain  SubClassName=ps_output  LeftPortType=input  RightPortType=output  PseudoPeriodic=off  Frequencies=[]  VectorFormat=inherit  Unit=inherit  AffineConversion=off
  Simulink-PS Converter : nesl_utility/Simulink-PS Converter  PhysicalDomain=network_engine_domain  SubClassName=ps_input  LeftPortType=input  RightPortType=output  PseudoPeriodic=off  Frequencies=[]  NoiseDistribution=none  NoiseParameters=[]  Unit=1  AffineConversion=off  FilteringAndDerivatives=provide  SimscapeFilterOrder=1  InputFilterTimeConstant=0.001  UdotUserProvided=0
  Transform Sensor : sm_lib/Frames and Transforms/Transform Sensor  MeasurementFrame=World  SenseAngle=off  SenseAxis=off  SenseQ=off  SenseR=off  SenseRotationSequence=off  RotationSequence=XYX  SenseOmegaX=off  SenseOmegaY=off  SenseOmegaZ=off  SenseQDot=off  SenseRDot=off  SenseAlphaX=off  SenseAlphaY=off  SenseAlphaZ=off  SenseQDDot=off  SenseRDDot=off  SenseX=off  SenseY=off  SenseZ=off  SenseRad=off  SenseAzim=off  SenseDist=on  SenseInc=off  SenseXDot=off  SenseYDot=off  SenseZDot=off  SenseRadDot=off  SenseAzimDot=off  SenseDistDot=on  SenseIncDot=off  SenseXDDot=off  SenseYDDot=off  SenseZDDot=off  SenseRadDDot=off  SenseAzimDDot=off  SenseDistDDot=off  SenseIncDDot=off
  cable force : MATLAB Function  TreatAsAtomicUnit=on
  l : Display
  l0 : Display
  v : Display
  bar_point_bown : PMIOPort  Side=Left
  bar_point_up : PMIOPort  Port=2  Side=Right
  wires:
  cable force/1(Fl) -> Gain/1
  PS-Simulink Converter/1 -> l/1
  Constant2/1 -> MATLAB Function/4(l0)
  MATLAB Function/2(bi) -> cable force/2(b)
  Constant1/1 -> MATLAB Function/3(bb)
  Constant/1 -> MATLAB Function/2(kk)
  MATLAB Function/1(ki) -> cable force/1(k)
  PS-Simulink Converter1/1 -> cable force/4(l)
  MATLAB Function/3(l0i) -> l0/1, cable force/3(l0)
  i/1 -> MATLAB Function/1(i)
  Constant3/1 -> cable force/6(bar_or_cable)
  Gain/1 -> Simulink-PS Converter/1
  PS-Simulink Converter2/1 -> cable force/5(v)
  PS-Simulink Converter3/1 -> v/1
  connections:
  Internal Force/LConn1 -- bar_point_bown/RConn1
  PS-Simulink Converter/LConn1 -- Transform Sensor/RConn2 -- PS-Simulink Converter1/LConn1
  Simulink-PS Converter/RConn1 -- Internal Force/LConn2
  Internal Force/RConn1 -- Transform Sensor/RConn1 -- bar_point_up/RConn1
  Connection Label1/LConn1 -- Transform Sensor/LConn1
  PS-Simulink Converter2/LConn1 -- Transform Sensor/RConn3 -- PS-Simulink Converter3/LConn1

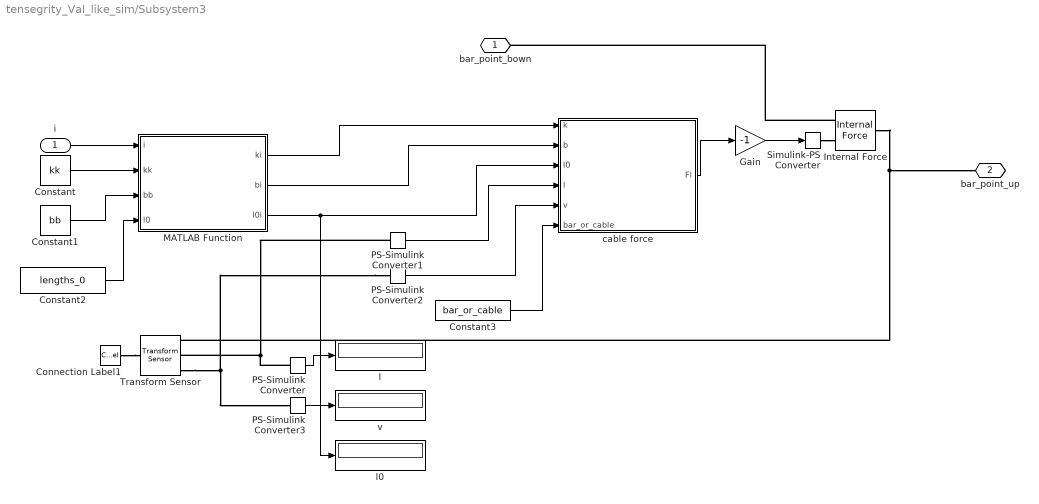
== system tensegrity_Val_like_sim/Subsystem3 ==
  i : Inport
  Connection Label1 : ConnectionLabel  Label=base_frame
  Constant : Constant  Value=kk
  Constant1 : Constant  Value=bb
  Constant2 : Constant  Value=lengths_0
  Constant3 : Constant  Value=bar_or_cable
  Gain : Gain  Gain=-1
  Internal Force : sm_lib/Forces and Torques/Internal Force
  MATLAB Function : MATLAB Function  TreatAsAtomicUnit=on
  PS-Simulink Converter{,1..3} (4 alike) : nesl_utility/PS-Simulink Converter  PhysicalDomain=network_engine_domain  SubClassName=ps_output  LeftPortType=input  RightPortType=output  PseudoPeriodic=off  Frequencies=[]  VectorFormat=inherit  Unit=inherit  AffineConversion=off
  Simulink-PS Converter : nesl_utility/Simulink-PS Converter  PhysicalDomain=network_engine_domain  SubClassName=ps_input  LeftPortType=input  RightPortType=output  PseudoPeriodic=off  Frequencies=[]  NoiseDistribution=none  NoiseParameters=[]  Unit=1  AffineConversion=off  FilteringAndDerivatives=provide  SimscapeFilterOrder=1  InputFilterTimeConstant=0.001  UdotUserProvided=0
  Transform Sensor : sm_lib/Frames and Transforms/Transform Sensor  MeasurementFrame=World  SenseAngle=off  SenseAxis=off  SenseQ=off  SenseR=off  SenseRotationSequence=off  RotationSequence=XYX  SenseOmegaX=off  SenseOmegaY=off  SenseOmegaZ=off  SenseQDot=off  SenseRDot=off  SenseAlphaX=off  SenseAlphaY=off  SenseAlphaZ=off  SenseQDDot=off  SenseRDDot=off  SenseX=off  SenseY=off  SenseZ=off  SenseRad=off  SenseAzim=off  SenseDist=on  SenseInc=off  SenseXDot=off  SenseYDot=off  SenseZDot=off  SenseRadDot=off  SenseAzimDot=off  SenseDistDot=on  SenseIncDot=off  SenseXDDot=off  SenseYDDot=off  SenseZDDot=off  SenseRadDDot=off  SenseAzimDDot=off  SenseDistDDot=off  SenseIncDDot=off
  cable force : MATLAB Function  TreatAsAtomicUnit=on
  l : Display
  l0 : Display
  v : Display
  bar_point_bown : PMIOPort  Side=Left
  bar_point_up : PMIOPort  Port=2  Side=Right
  wires:
  cable force/1(Fl) -> Gain/1
  PS-Simulink Converter/1 -> l/1
  Constant2/1 -> MATLAB Function/4(l0)
  MATLAB Function/2(bi) -> cable force/2(b)
  Constant1/1 -> MATLAB Function/3(bb)
  Constant/1 -> MATLAB Function/2(kk)
  MATLAB Function/1(ki) -> cable force/1(k)
  PS-Simulink Converter1/1 -> cable force/4(l)
  MATLAB Function/3(l0i) -> l0/1, cable force/3(l0)
  i/1 -> MATLAB Function/1(i)
  Constant3/1 -> cable force/6(bar_or_cable)
  Gain/1 -> Simulink-PS Converter/1
  PS-Simulink Converter2/1 -> cable force/5(v)
  PS-Simulink Converter3/1 -> v/1
  connections:
  Internal Force/LConn1 -- bar_point_bown/RConn1
  PS-Simulink Converter/LConn1 -- Transform Sensor/RConn2 -- PS-Simulink Converter1/LConn1
  Simulink-PS Converter/RConn1 -- Internal Force/LConn2
  Internal Force/RConn1 -- Transform Sensor/RConn1 -- bar_point_up/RConn1
  Connection Label1/LConn1 -- Transform Sensor/LConn1
  PS-Simulink Converter2/LConn1 -- Transform Sensor/RConn3 -- PS-Simulink Converter3/LConn1

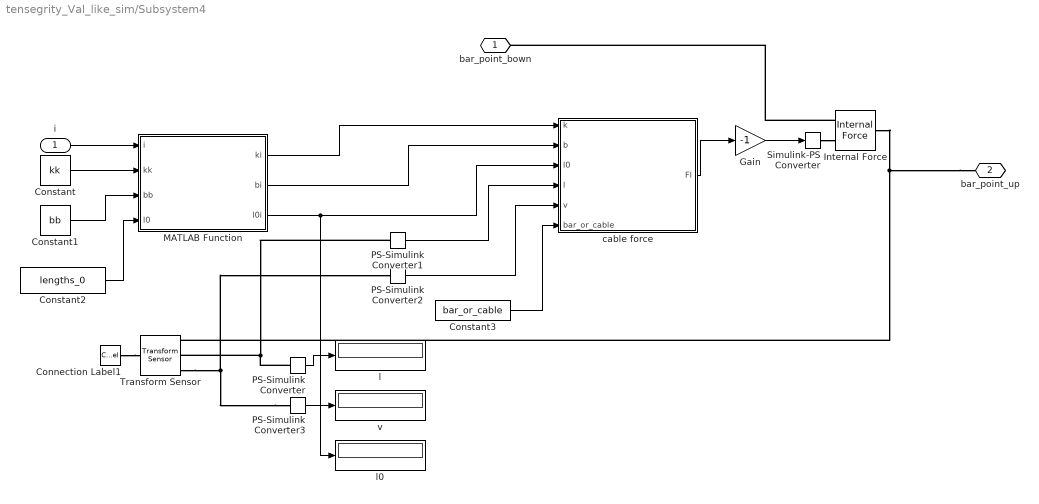
== system tensegrity_Val_like_sim/Subsystem4 ==
  i : Inport
  Connection Label1 : ConnectionLabel  Label=base_frame
  Constant : Constant  Value=kk
  Constant1 : Constant  Value=bb
  Constant2 : Constant  Value=lengths_0
  Constant3 : Constant  Value=bar_or_cable
  Gain : Gain  Gain=-1
  Internal Force : sm_lib/Forces and Torques/Internal Force
  MATLAB Function : MATLAB Function  TreatAsAtomicUnit=on
  PS-Simulink Converter{,1..3} (4 alike) : nesl_utility/PS-Simulink Converter  PhysicalDomain=network_engine_domain  SubClassName=ps_output  LeftPortType=input  RightPortType=output  PseudoPeriodic=off  Frequencies=[]  VectorFormat=inherit  Unit=inherit  AffineConversion=off
  Simulink-PS Converter : nesl_utility/Simulink-PS Converter  PhysicalDomain=network_engine_domain  SubClassName=ps_input  LeftPortType=input  RightPortType=output  PseudoPeriodic=off  Frequencies=[]  NoiseDistribution=none  NoiseParameters=[]  Unit=1  AffineConversion=off  FilteringAndDerivatives=provide  SimscapeFilterOrder=1  InputFilterTimeConstant=0.001  UdotUserProvided=0
  Transform Sensor : sm_lib/Frames and Transforms/Transform Sensor  MeasurementFrame=World  SenseAngle=off  SenseAxis=off  SenseQ=off  SenseR=off  SenseRotationSequence=off  RotationSequence=XYX  SenseOmegaX=off  SenseOmegaY=off  SenseOmegaZ=off  SenseQDot=off  SenseRDot=off  SenseAlphaX=off  SenseAlphaY=off  SenseAlphaZ=off  SenseQDDot=off  SenseRDDot=off  SenseX=off  SenseY=off  SenseZ=off  SenseRad=off  SenseAzim=off  SenseDist=on  SenseInc=off  SenseXDot=off  SenseYDot=off  SenseZDot=off  SenseRadDot=off  SenseAzimDot=off  SenseDistDot=on  SenseIncDot=off  SenseXDDot=off  SenseYDDot=off  SenseZDDot=off  SenseRadDDot=off  SenseAzimDDot=off  SenseDistDDot=off  SenseIncDDot=off
  cable force : MATLAB Function  TreatAsAtomicUnit=on
  l : Display
  l0 : Display
  v : Display
  bar_point_bown : PMIOPort  Side=Left
  bar_point_up : PMIOPort  Port=2  Side=Right
  wires:
  PS-Simulink Converter3/1 -> v/1
  PS-Simulink Converter2/1 -> cable force/5(v)
  Gain/1 -> Simulink-PS Converter/1
  Constant3/1 -> cable force/6(bar_or_cable)
  i/1 -> MATLAB Function/1(i)
  MATLAB Function/3(l0i) -> cable force/3(l0), l0/1
  PS-Simulink Converter1/1 -> cable force/4(l)
  MATLAB Function/1(ki) -> cable force/1(k)
  Constant/1 -> MATLAB Function/2(kk)
  Constant1/1 -> MATLAB Function/3(bb)
  MATLAB Function/2(bi) -> cable force/2(b)
  Constant2/1 -> MATLAB Function/4(l0)
  PS-Simulink Converter/1 -> l/1
  cable force/1(Fl) -> Gain/1
  connections:
  PS-Simulink Converter3/LConn1 -- Transform Sensor/RConn3 -- PS-Simulink Converter2/LConn1
  Connection Label1/LConn1 -- Transform Sensor/LConn1
  bar_point_up/RConn1 -- Transform Sensor/RConn1 -- Internal Force/RConn1
  Simulink-PS Converter/RConn1 -- Internal Force/LConn2
  PS-Simulink Converter1/LConn1 -- Transform Sensor/RConn2 -- PS-Simulink Converter/LConn1
  Internal Force/LConn1 -- bar_point_bown/RConn1

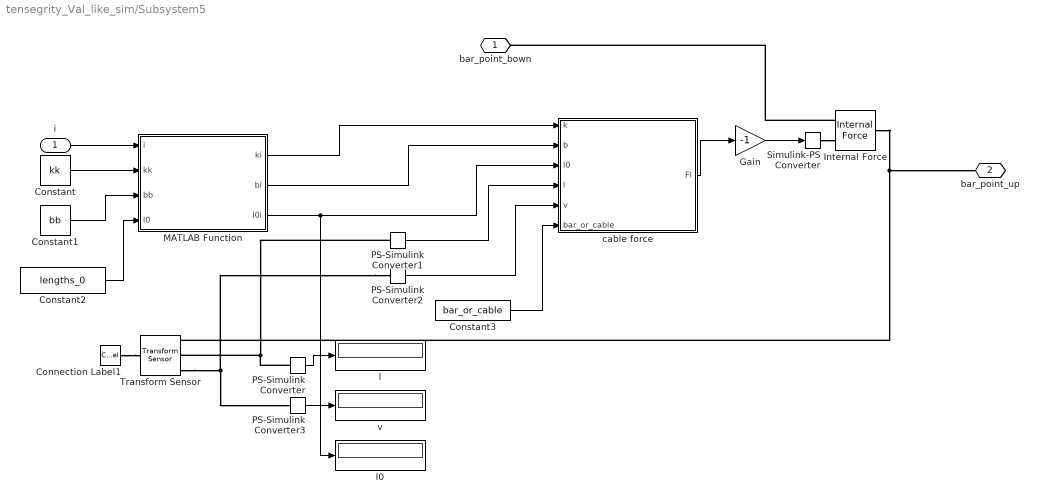
== system tensegrity_Val_like_sim/Subsystem5 ==
  i : Inport
  Connection Label1 : ConnectionLabel  Label=base_frame
  Constant : Constant  Value=kk
  Constant1 : Constant  Value=bb
  Constant2 : Constant  Value=lengths_0
  Constant3 : Constant  Value=bar_or_cable
  Gain : Gain  Gain=-1
  Internal Force : sm_lib/Forces and Torques/Internal Force
  MATLAB Function : MATLAB Function  TreatAsAtomicUnit=on
  PS-Simulink Converter{,1..3} (4 alike) : nesl_utility/PS-Simulink Converter  PhysicalDomain=network_engine_domain  SubClassName=ps_output  LeftPortType=input  RightPortType=output  PseudoPeriodic=off  Frequencies=[]  VectorFormat=inherit  Unit=inherit  AffineConversion=off
  Simulink-PS Converter : nesl_utility/Simulink-PS Converter  PhysicalDomain=network_engine_domain  SubClassName=ps_input  LeftPortType=input  RightPortType=output  PseudoPeriodic=off  Frequencies=[]  NoiseDistribution=none  NoiseParameters=[]  Unit=1  AffineConversion=off  FilteringAndDerivatives=provide  SimscapeFilterOrder=1  InputFilterTimeConstant=0.001  UdotUserProvided=0
  Transform Sensor : sm_lib/Frames and Transforms/Transform Sensor  MeasurementFrame=World  SenseAngle=off  SenseAxis=off  SenseQ=off  SenseR=off  SenseRotationSequence=off  RotationSequence=XYX  SenseOmegaX=off  SenseOmegaY=off  SenseOmegaZ=off  SenseQDot=off  SenseRDot=off  SenseAlphaX=off  SenseAlphaY=off  SenseAlphaZ=off  SenseQDDot=off  SenseRDDot=off  SenseX=off  SenseY=off  SenseZ=off  SenseRad=off  SenseAzim=off  SenseDist=on  SenseInc=off  SenseXDot=off  SenseYDot=off  SenseZDot=off  SenseRadDot=off  SenseAzimDot=off  SenseDistDot=on  SenseIncDot=off  SenseXDDot=off  SenseYDDot=off  SenseZDDot=off  SenseRadDDot=off  SenseAzimDDot=off  SenseDistDDot=off  SenseIncDDot=off
  cable force : MATLAB Function  TreatAsAtomicUnit=on
  l : Display
  l0 : Display
  v : Display
  bar_point_bown : PMIOPort  Side=Left
  bar_point_up : PMIOPort  Port=2  Side=Right
  wires:
  cable force/1(Fl) -> Gain/1
  PS-Simulink Converter/1 -> l/1
  Constant2/1 -> MATLAB Function/4(l0)
  MATLAB Function/2(bi) -> cable force/2(b)
  Constant1/1 -> MATLAB Function/3(bb)
  Constant/1 -> MATLAB Function/2(kk)
  MATLAB Function/1(ki) -> cable force/1(k)
  PS-Simulink Converter1/1 -> cable force/4(l)
  MATLAB Function/3(l0i) -> l0/1, cable force/3(l0)
  i/1 -> MATLAB Function/1(i)
  Constant3/1 -> cable force/6(bar_or_cable)
  Gain/1 -> Simulink-PS Converter/1
  PS-Simulink Converter2/1 -> cable force/5(v)
  PS-Simulink Converter3/1 -> v/1
  connections:
  Internal Force/LConn1 -- bar_point_bown/RConn1
  PS-Simulink Converter/LConn1 -- Transform Sensor/RConn2 -- PS-Simulink Converter1/LConn1
  Simulink-PS Converter/RConn1 -- Internal Force/LConn2
  Internal Force/RConn1 -- Transform Sensor/RConn1 -- bar_point_up/RConn1
  Connection Label1/LConn1 -- Transform Sensor/LConn1
  PS-Simulink Converter2/LConn1 -- Transform Sensor/RConn3 -- PS-Simulink Converter3/LConn1

== matlab function tensegrity_Val_like_sim/Subsystem4/MATLAB Function ==
  data: i input; ki output; kk input; bb input; l0 input; bi output; l0i output
function [ki, bi, l0i] = parameter_selection(i, kk, bb, l0)

l0i=l0(i);
ki=kk;
bi=bb;

== matlab function tensegrity_Val_like_sim/Subsystem/MATLAB Function ==
  data: i input; ki output; kk input; bb input; l0 input; bi output; l0i output
function [ki, bi, l0i] = parameter_selection(i, kk, bb, l0)

l0i=l0(i);
ki=kk;
bi=bb;

== matlab function tensegrity_Val_like_sim/Subsystem4/cable force ==
  data: k input; Fl output; b input; l0 input; l input; v input; bar_or_cable input
function Fl = fcn(k, b, l0, l, v, bar_or_cable)

Fl=0; %if not bar, but cable only

l-l0

if(l>l0)
  Fl=k*(l-l0) + v*b;
end;

if(bar_or_cable==1) % if bar==1, the force can act in both directions
  Fl=k*(l-l0) + v*b;
end;

== matlab function tensegrity_Val_like_sim/Subsystem5/MATLAB Function ==
  data: i input; ki output; kk input; bb input; l0 input; bi output; l0i output
function [ki, bi, l0i] = parameter_selection(i, kk, bb, l0)

l0i=l0(i);
ki=kk;
bi=bb;

== matlab function tensegrity_Val_like_sim/Subsystem5/cable force ==
  data: k input; Fl output; b input; l0 input; l input; v input; bar_or_cable input
function Fl = fcn(k, b, l0, l, v, bar_or_cable)

Fl=0; %if not bar, but cable only

l-l0

if(l>l0)
  Fl=k*(l-l0) + v*b;
end;

if(bar_or_cable==1) % if bar==1, the force can act in both directions
  Fl=k*(l-l0) + v*b;
end;

== matlab function tensegrity_Val_like_sim/Subsystem/cable force ==
  data: k input; Fl output; b input; l0 input; l input; v input; bar_or_cable input
function Fl = fcn(k, b, l0, l, v, bar_or_cable)

Fl=0; %if not bar, but cable only

l-l0

if(l>l0)
  Fl=k*(l-l0) + v*b;
end;

if(bar_or_cable==1) % if bar==1, the force can act in both directions
  Fl=k*(l-l0) + v*b;
end;

== matlab function tensegrity_Val_like_sim/Subsystem1/MATLAB Function ==
  data: i input; ki output; kk input; bb input; l0 input; bi output; l0i output
function [ki, bi, l0i] = parameter_selection(i, kk, bb, l0)

l0i=l0(i);
ki=kk;
bi=bb;

== matlab function tensegrity_Val_like_sim/Subsystem1/cable force ==
  data: k input; Fl output; b input; l0 input; l input; v input; bar_or_cable input
function Fl = fcn(k, b, l0, l, v, bar_or_cable)

Fl=0; %if not bar, but cable only

l-l0

if(l>l0)
  Fl=k*(l-l0) + v*b;
end;

if(bar_or_cable==1) % if bar==1, the force can act in both directions
  Fl=k*(l-l0) + v*b;
end;

== matlab function tensegrity_Val_like_sim/Subsystem2/MATLAB Function ==
  data: i input; ki output; kk input; bb input; l0 input; bi output; l0i output
function [ki, bi, l0i] = parameter_selection(i, kk, bb, l0)

l0i=l0(i);
ki=kk;
bi=bb;

== matlab function tensegrity_Val_like_sim/Subsystem2/cable force ==
  data: k input; Fl output; b input; l0 input; l input; v input; bar_or_cable input
function Fl = fcn(k, b, l0, l, v, bar_or_cable)

Fl=0; %if not bar, but cable only

l-l0

if(l>l0)
  Fl=k*(l-l0) + v*b;
end;

if(bar_or_cable==1) % if bar==1, the force can act in both directions
  Fl=k*(l-l0) + v*b;
end;

== matlab function tensegrity_Val_like_sim/Subsystem3/MATLAB Function ==
  data: i input; ki output; kk input; bb input; l0 input; bi output; l0i output
function [ki, bi, l0i] = parameter_selection(i, kk, bb, l0)

l0i=l0(i);
ki=kk;
bi=bb;

== matlab function tensegrity_Val_like_sim/Subsystem3/cable force ==
  data: k input; Fl output; b input; l0 input; l input; v input; bar_or_cable input
function Fl = fcn(k, b, l0, l, v, bar_or_cable)

Fl=0; %if not bar, but cable only

l-l0

if(l>l0)
  Fl=k*(l-l0) + v*b;
end;

if(bar_or_cable==1) % if bar==1, the force can act in both directions
  Fl=k*(l-l0) + v*b;
end;
